simulink subsystem "speed_error_sub"  (R2025b)
settings: Solver=VariableStepAuto  StartTime=0.0  StopTime=10.0  RelTol=1e-3
libraries: simulink x1
settings Model: Creator=erik  LastModifiedBy=erik

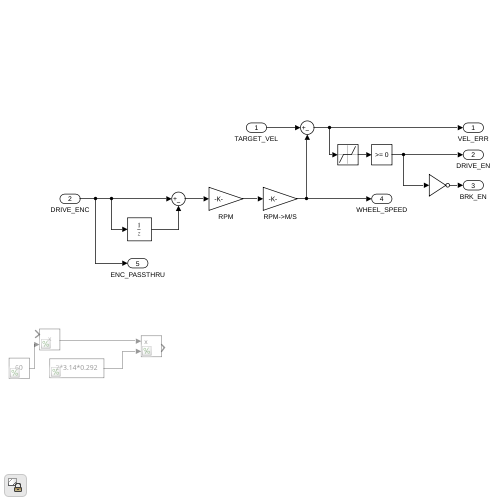
[thumbnail: Simulink's stored preview of the top-level diagram]
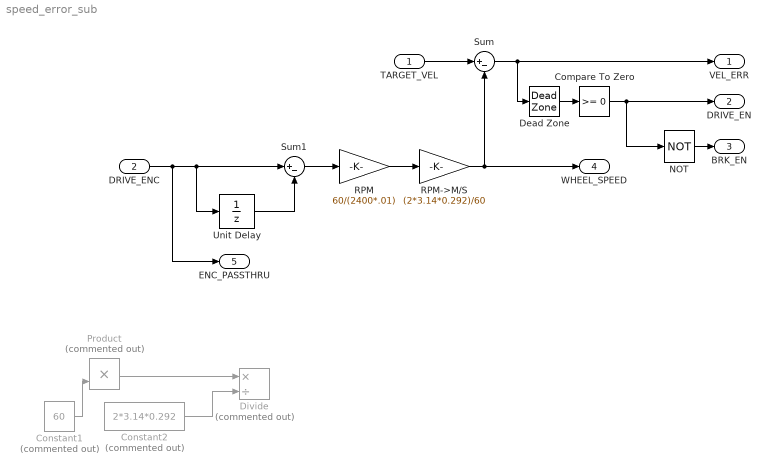
== system speed_error_sub ==
  TARGET_VEL : Inport
  DRIVE_ENC : Inport  Port=2
  Compare To Zero : simulink/Logic and Bit Operations/Compare To Zero  relop=>=  OutDataTypeStr=boolean
  Constant1 : Constant  Commented=on  Value=60
  Constant2 : Constant  Commented=on  Value=2*3.14*0.292
  Dead Zone : DeadZone  LowerValue=-1.0  UpperValue=0.0
  Divide : Product  Commented=on  Inputs=*/
  NOT : Logic  Operator=NOT  IconShape=distinctive  AllPortsSameDT=off  OutDataTypeStr=boolean
  Product : Product  Commented=on
  RPM : Gain  Gain=60/(2400*.01)
  RPM->M/S : Gain  Gain=(2*3.14*0.292)/60  OutDataTypeStr=single
  Sum : Sum  Inputs=|+-
  Sum1 : Sum  Inputs=|+-
  Unit Delay : UnitDelay  SampleTime=.01  HasFrameUpgradeWarning=on
  VEL_ERR : Outport
  DRIVE_EN : Outport  Port=2
  BRK_EN : Outport  Port=3
  WHEEL_SPEED : Outport  Port=4
  ENC_PASSTHRU : Outport  Port=5
  wires:
  Constant2/1 -> Divide/2
  Unit Delay/1 -> Sum1/2
  Product/1 -> Divide/1
  DRIVE_ENC/1 -> Sum1/1, Unit Delay/1, ENC_PASSTHRU/1
  Constant1/1 -> Product/2
  Dead Zone/1 -> Compare To Zero/1
  NOT/1 -> BRK_EN/1
  Sum/1 -> VEL_ERR/1, Dead Zone/1
  RPM/1 -> RPM->M/S/1
  RPM->M/S/1 -> Sum/2, WHEEL_SPEED/1
  TARGET_VEL/1 -> Sum/1
  Sum1/1 -> RPM/1
  Compare To Zero/1 -> DRIVE_EN/1, NOT/1
